simulink model "computedTorqueControlV2"  (R2014b)
settings: Solver=FixedStepDiscrete  StartTime=0.0  StopTime=simulationTime  FixedStep=Ts  RelTol=1e-3
InitFcn:
  | init_computedTorqueControlV2;
values from neighbouring files (symbols this model uses):
  ampl_and_freq = [ 20 ... (first row only)    [init_computedTorqueControl.m]    (also in init_computedTorqueControlV2.m)
  Kd = 2*sqrt(Kp)    [init_computedTorqueControl.m]    (also in init_computedTorqueControlV2.m)
  Kp = 70*diag( ones(1,ROBOT_DOF)  )    [init_computedTorqueControl.m]    (also in init_computedTorqueControlV2.m = 250*diag( ones(1,ROBOT_DOF)  ))
  ROBOT_DOF = 1    [init_computedTorqueControl.m]    (also in init_computedTorqueControlV2.m)
  Ts = 0.01    [init_computedTorqueControl.m]    (also in init_computedTorqueControlV2.m)
libraries: WBCLibrary x9
settings Model: Creator=daniele  LastModifiedBy=pucci
settings DataIOCC: SignalLoggingSaveFormat=ModelDataLogs
settings DebuggingCC: MultiTaskDSMMsg=warning  MultiTaskCondExecSysMsg=none  StrictBusMsg=ErrorOnBusTreatedAsVector
settings RTWCC: IncludeERTFirstTime=on

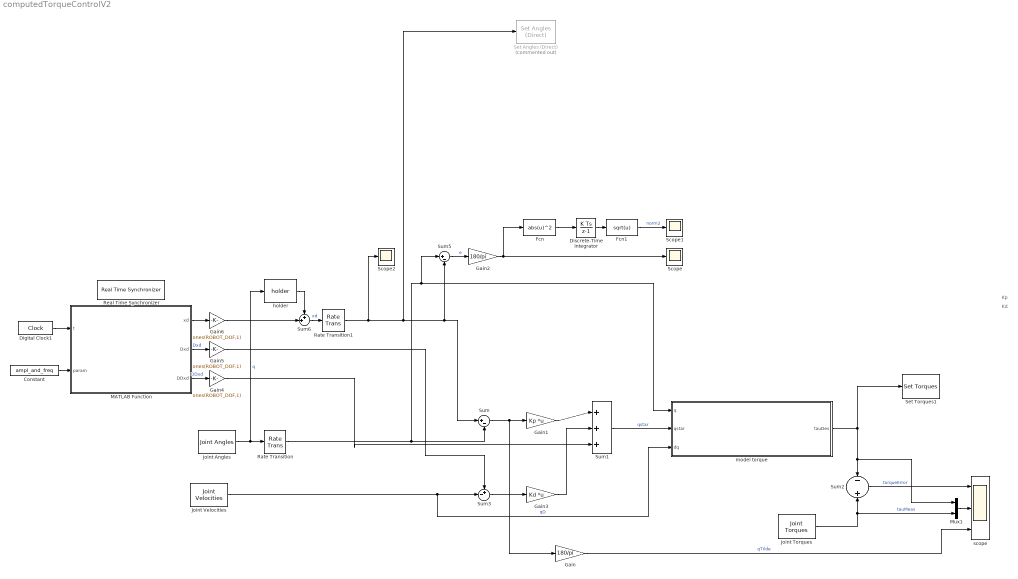
== system computedTorqueControlV2 ==
  note: Kd
  note: Kp
  Constant : Constant  Value=ampl_and_freq
  Digital Clock1 : DigitalClock  SampleTime=Ts
  Discrete-Time Integrator : DiscreteIntegrator  InitialConditionSetting=State (most efficient)  SampleTime=Ts
  Fcn : Fcn  Expr=abs(u)^2
  Fcn1 : Fcn  Expr=sqrt(u)
  Gain : Gain  Gain=180/pi
  Gain1 : Gain  Gain=Kp  Multiplication=Matrix(K*u)
  Gain2 : Gain  Gain=180/pi
  Gain3 : Gain  Gain=Kd  Multiplication=Matrix(K*u)
  Gain4 : Gain  Gain=ones(ROBOT_DOF,1)
  Gain5 : Gain  Gain=ones(ROBOT_DOF,1)  SampleTime=Ts
  Gain6 : Gain  Gain=ones(ROBOT_DOF,1)  SampleTime=Ts
  Joint Angles : WBCLibrary/wholeBodyStates/Joint Angles  robotName=robotName  localName=localName
  Joint Torques : WBCLibrary/wholeBodyStates/Joint Torques  robotName=robotName  localName=localName
  Joint Velocities : WBCLibrary/wholeBodyStates/Joint Velocities  robotName=robotName  localName=localName
  MATLAB Function : MATLAB Function  TreatAsAtomicUnit=on
  Mux1 : Mux  Inputs=2
  Rate Transition : RateTransition  OutPortSampleTime=Ts
  Rate Transition1 : RateTransition  OutPortSampleTime=Ts
  Real Time Synchronizer : WBCLibrary/Utilities/Real Time Synchronizer  Priority=-10  threadPeriod=Ts
  Scope : Scope
      settings: TimeRange=12.5  YMin=-6  YMax=8  SaveName=ScopeData2
  Scope1 : Scope
      settings: TimeRange=12.5  YMin=0  YMax=0.07000000000000001  SaveName=ScopeData3
  Scope2 : Scope
      settings: SaveName=ScopeData4
  Set Angles (Direct) : WBCLibrary/wholeBodyActuators/Set Angles (Direct)  Commented=on  val=20  robotName=robotName  localName=localName
  Set Torques1 : WBCLibrary/wholeBodyActuators/Set Torques  val=6  robotName=robotName  localName=localName
  Sum : Sum  Inputs=|+-
  Sum1 : Sum  Inputs=|+++
  Sum2 : Sum  Inputs=-|+
  Sum3 : Sum  Inputs=+-|
  Sum5 : Sum  Inputs=|+-
  Sum6 : Sum  Inputs=++|
  "holder " : WBCLibrary/Utilities/holder 
  model torque : Subsystem
  scope : Scope  NumInputPorts=3
      settings: ShowLegends=on  TimeRange=12.5  YMin=-25~-20~-2  YMax=25~30~4
  wires:
  Digital Clock1/1 -> MATLAB Function/1(t)
  Constant/1 -> MATLAB Function/2(param)
  Sum6/1 -> Rate Transition1/1  "xd"
  Gain1/1 -> Sum1/1
  Joint Torques/1 -> Mux1/2, Sum2/2  "tauMeas"
  Sum2/1 -> scope/1  "torqueError"
  Mux1/1 -> scope/2
  Sum/1 -> Gain1/1, Gain/1
  Sum3/1 -> Gain3/1
  MATLAB Function/2(Dxd) -> Gain5/1  "Dxd"
  Gain3/1 -> Sum1/2
  Gain/1 -> scope/3  "qTilde"
  MATLAB Function/3(DDxd) -> Gain4/1  "DDxd"
  Joint Velocities/1 -> Sum3/2, model torque/3(dq)  "qD"
  Sum5/1 -> Gain2/1  "e"
  Fcn/1 -> Discrete-Time Integrator/1
  Joint Angles/1 -> Rate Transition/1, "holder "/1  "q"
  Gain2/1 -> Fcn/1, Scope/1
  Rate Transition/1 -> Sum/2, Sum5/1, model torque/1(q)
  Fcn1/1 -> Scope1/1  "norm2"
  Discrete-Time Integrator/1 -> Fcn1/1
  "holder "/1 -> Sum6/1
  MATLAB Function/1(xd) -> Gain6/1
  Rate Transition1/1 -> Scope2/1, Set Angles (Direct)/1, Sum/1, Sum5/2
  Gain6/1 -> Sum6/2
  Gain5/1 -> Sum3/1
  Gain4/1 -> Sum1/3
  model torque/1(tauDes) -> Set Torques1/1, Mux1/1, Sum2/1
  Sum1/1 -> model torque/2(qstar)  "qstar"

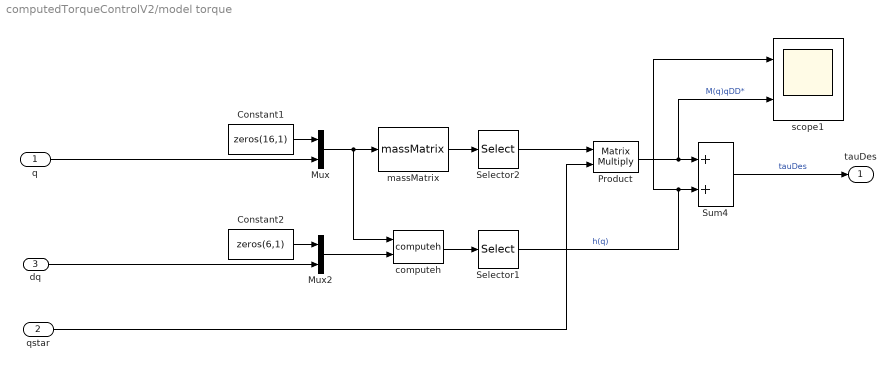
== system computedTorqueControlV2/model torque ==
  q : Inport
  qstar : Inport  Port=2
  dq : Inport  Port=3
  Constant1 : Constant  Value=zeros(16,1)
  Constant2 : Constant  Value=zeros(6,1)
  Mux : Mux  Inputs=2
  Mux2 : Mux  Inputs=2
  Product : Product  Multiplication=Matrix(*)
  Selector1 : Selector  InputPortWidth=ROBOT_DOF+6  Indices=[7:ROBOT_DOF+6]
  Selector2 : Selector  NumberOfDimensions=2  InputPortWidth=ROBOT_DOF+6  IndexOptions=Index vector (dialog),Index vector (dialog)  Indices=[7:6+ROBOT_DOF],[7:6+ROBOT_DOF]  OutputSizes=1,1
  Sum4 : Sum
  computeh : WBCLibrary/wholeBodyModel/Dynamics/computeh  val=7  robotname=robotName  localname=localName
  massMatrix : WBCLibrary/wholeBodyModel/Dynamics/massMatrix  val=8  robotname=robotName  localname=localName
  scope1 : Scope  NumInputPorts=2
      settings: ShowLegends=on  TimeRange=20  YMin=-8~-6  YMax=8~8
  tauDes : Outport
  wires:
  Selector1/1 -> scope1/1, Sum4/2  "h(q)"
  Sum4/1 -> tauDes/1  "tauDes"
  massMatrix/1 -> Selector2/1
  Product/1 -> Sum4/1, scope1/2  "M(q)qDD*"
  Selector2/1 -> Product/1
  qstar/1 -> Product/2
  Constant2/1 -> Mux2/1
  Mux2/1 -> computeh/2
  computeh/1 -> Selector1/1
  Mux/1 -> computeh/1, massMatrix/1
  Constant1/1 -> Mux/1
  dq/1 -> Mux2/2
  q/1 -> Mux/2

== matlab function computedTorqueControlV2/MATLAB Function ==
  data: t input; xd output; param input; Dxd output; DDxd output
function [xd,Dxd,DDxd] = fcn(t,param)
%#codegen

xd =  param(1)*sin(param(2)*t);

Dxd =  param(1)*param(2)*cos(param(2)*t);

DDxd = -param(1)*param(2)^2*sin(param(2)*t);
